simulink model "Quaternions_Method_merge"  (R2021b)
settings: Solver=VariableStepAuto  StartTime=0.0  StopTime=Time  FixedStep=1e-1  RelTol=1e-13  AbsTol=1e-8
values from neighbouring files (symbols this model uses):
  a = 8.6251e+06    (= 8625100)    [Main.m]    (also in main_code.m)
  A_rw = [1 0 0 1/sqrt(3);         0 1 0 1/sqrt(3) ... (first row only)    [Main.m]    (also in main_code.m)
  A_rw_star = [5/6 -1/6 -1/6;              -1/6  5/6 -1/6 ... (first row only)    [Main.m]    (also in main_code.m)
  c = 299792*10^3    (= 299792000)    [Main.m]    (also in main_code.m)
  e = 0.1195    [Main.m]    (also in main_code.m)
  f_mag = 5    [Main.m]
  H_0 = sqrt((g_1_0)^2 + (g_1_1)^2 + (h_1_1)^2)    [Main.m]
  i = 0.3815    [Main.m]    (also in main_code.m)
  MB = [2000; 0.3; 1; 0.12].*1e-2    [Main.m]    (also in main_code.m = [1; 0.3; 0.3; 0.3])
  mr = 1.2*1e-4    (= 0.00012)    [Main.m]    (also in main_code.m)
  muP = G*Mt    (= 398527110340000)    [Main.m]
  omega_0 = [om_x, om_y, om_z]    [Main.m]    (also in main_code.m = [w_0x; w_0y; w_0z])
  p_acc = deg2rad(5)    [Main.m]
  RD = 0.1*ones(1,10)    [Main.m]
  RS_MB = 0.5    [Main.m]
  RS_SP = 0.1    [Main.m]
  sig_b = sig_b^2    [Main.m]    (also in main_code.m)
  sig_n = 0.15*pi/180/3600/sqrt(t_sample)    [Main.m]    (also in main_code.m)
  SP = [2000; 0.3; 1; 0.12].*1e-2    [Main.m]    (also in main_code.m = [3; 0.3; 1; 0.1])
  T = 2*pi/n    [Main.m]    (also in main_code.m = 2*pi / n)
  t_sample = 1/5    (= 0.2)    [Main.m]    (also in main_code.m = 0.1)
  theta0 = 0    [Main.m]
  w_E = (2*pi)/(24*3600)    (= 7.27220521664e-05)    [Main.m]
undefined symbols (not defined in the file or in its folder): magnitude
libraries: matrix_library x14, vrlib x8, simulink x2, simulink_extras x1
(part 2 of 4)

== system Quaternions_Method_merge/Kinematics/Relative_Attitude ==
  A_BN : Inport
  theta : Inport  Port=2
  A_LN : Subsystem
  MatrixMultiply : Product  Multiplication=Matrix(*)
  Transpose : Math  Operator=transpose  SaturateOnIntegerOverflow=on
  A_BL : Outport
  A_L/N : Outport  Port=2
  wires:
  Transpose/1 -> MatrixMultiply/2
  MatrixMultiply/1 -> A_BL/1  "A_BL"
  A_LN/1(A_LN) -> Transpose/1, A_L/N/1
  A_BN/1 -> MatrixMultiply/1
  theta/1 -> A_LN/1(theta)

== system Quaternions_Method_merge/Sensors/Gyroscopes ==
  note: gyro model: STIM300
  omega : Inport
  Integrator : Integrator
  Mux1 : Mux  Inputs=3
  Mux2 : Mux  Inputs=3
  Reshape : Reshape  OutputDimensionality=Column vector (2-D)
  Reshape1 : Reshape  OutputDimensionality=Column vector (2-D)
  Sum : Sum  Inputs=+++
  "b1 " : RandomNumber  Variance=sig_b  Seed=1  SampleTime=t_sample
  b2 : RandomNumber  Variance=sig_b  Seed=2  SampleTime=t_sample
  b3 : RandomNumber  Variance=sig_b  Seed=3  SampleTime=t_sample
  n1 : RandomNumber  Variance=sig_n  Seed=4  SampleTime=t_sample
  n2 : RandomNumber  Variance=sig_n  Seed=5  SampleTime=t_sample
  n3 : RandomNumber  Variance=sig_n  Seed=6  SampleTime=t_sample
  omega_m : Outport
  wires:
  Integrator/1 -> Sum/1
  "b1 "/1 -> Mux1/1
  b2/1 -> Mux1/2
  b3/1 -> Mux1/3
  n3/1 -> Mux2/3
  n2/1 -> Mux2/2
  n1/1 -> Mux2/1
  Mux1/1 -> Reshape/1
  Mux2/1 -> Reshape1/1
  Sum/1 -> omega_m/1
  omega/1 -> Sum/2
  Reshape/1 -> Integrator/1
  Reshape1/1 -> Sum/3

== system Quaternions_Method_merge/Sensors/Magnetometer1 ==
  A_BN : Inport
  b_N : Inport  Port=2
  "Magnetometer " : Subsystem
  b_B computation : Subsystem
  model to reality difference : Subsystem
  b_B : Outport
  wires:
  "Magnetometer "/1(A_BN*_filtered) -> b_B computation/1(A_BN*), model to reality difference/2(A_BN*)
  A_BN/1 -> model to reality difference/1(A_BN), "Magnetometer "/1(A_BN)
  b_N/1 -> b_B computation/2(b_N), model to reality difference/3(b_N)
  b_B computation/1(b_B) -> b_B/1
  "Magnetometer "/2(A_BN*_not_filtered) -> model to reality difference/4(A_BN*1)

== system Quaternions_Method_merge/Sensors/Sun sensor ==
  note: redwire space, digital sun sensor +/- 64°
  S_N : Inport
  A_BN : Inport  Port=2
  Add : Sum  Inputs=+-
  Add1 : Sum  Inputs=+-
  Constant : Constant  Value=0.25*pi/180
  Constant1 : Constant
  Constant2 : Constant  Value=0.25*pi/180
  Constant3 : Constant  Value=0.25*pi/180
  Delay1 : Delay  DelayLength=1
  Discrete Derivative : simulink/Discrete/Discrete Derivative  gainval=T^-1  ICPrevScaledInput=0.0  OutMin=[]  OutMax=[]  OutDataType=fixdt(1, 16)  OutScaling=2^-10  DoSatur=off
  Gain : Gain  Gain=-1
  Gain1 : Gain  Gain=-1
  Gain2 : Gain  Gain=-1
  Matrix Multiply : Product  Multiplication=Matrix(*)
  Matrix Multiply1 : Product  Multiplication=Matrix(*)
  Product : Product
  Product1 : Product
  Product2 : Product
  Random Number : RandomNumber  Variance=0.6*pi/180  SampleTime=1/1000
  Random Number1 : RandomNumber  Variance=0.6*pi/180  SampleTime=1/1000
  Random Number2 : RandomNumber  Variance=0.6*pi/180  SampleTime=1/1000
  Reshape : Reshape  OutputDimensionality=Customize  OutputDimensions=[3,3]
  Scope : Scope
  Vector Concatenate : Concatenate  NumInputs=9
  S_B : Outport
  wires:
  S_N/1 -> Matrix Multiply1/2
  Random Number/1 -> Product/2
  Constant/1 -> Product/1
  Matrix Multiply/1 -> Add1/1
  Discrete Derivative/1 -> Delay1/1
  Add1/1 -> Add/1, Discrete Derivative/1, S_B/1
  Constant1/1 -> Vector Concatenate/8, Vector Concatenate/5, Vector Concatenate/1
  Constant2/1 -> Product1/1
  Random Number1/1 -> Product1/2
  Random Number2/1 -> Product2/2
  Constant3/1 -> Product2/1
  Product2/1 -> Vector Concatenate/4, Gain/1
  Gain/1 -> Vector Concatenate/2
  Product1/1 -> Vector Concatenate/3, Gain2/1
  Gain1/1 -> Vector Concatenate/6
  Product/1 -> Gain1/1, Vector Concatenate/9
  Gain2/1 -> Vector Concatenate/7
  Delay1/1 -> Add1/2
  Reshape/1 -> Matrix Multiply/1
  Vector Concatenate/1 -> Reshape/1
  A_BN/1 -> Matrix Multiply1/1
  Matrix Multiply1/1 -> Add/2, Matrix Multiply/2
  Add/1 -> Scope/1

== system Quaternions_Method_merge/Sun Pointing /Pointing error with DCM ==
  A_B_N from attitude determination : Inport
  S_N : Inport  Port=2
  A_B_N from Euler : Inport  Port=3
  Add : Sum  Inputs=+|-
  Desired attitude : Subsystem
  Detected pointing error : Subsystem
  Real pointing error : Subsystem
  Difference between real and detected pointing error : Outport
  wires:
  A_B_N from attitude determination/1 -> Detected pointing error/2(A_B_N from attitude determination)
  Add/1 -> Difference between real and detected pointing error/1
  A_B_N from Euler/1 -> Real pointing error/1(" A_B_N from Euler")
  Desired attitude/1(Desired A_B_N) -> Real pointing error/2(Desired A_B_N), Detected pointing error/1(Desired A_B_N)
  Detected pointing error/1(detected pointing error) -> Add/2
  Real pointing error/1(real pointing error) -> Add/1
  S_N/1 -> Desired attitude/1(S_N)

== system Quaternions_Method_merge/Sun Pointing /Pointing error with quaternions ==
  A_B_N from attitude determination : Inport
  S_N : Inport  Port=2
  A_B_N from Euler : Inport  Port=3
  Add : Sum  Inputs=+|-
  Add1 : Sum  Inputs=+|-
  Creation of quaternion : Subsystem
  Creation of the quaternion : Subsystem
  Creation quaternion : Subsystem
  Desired attitude : Subsystem
  real pointing error : Outport
  detected pointing error : Outport  Port=2
  wires:
  S_N/1 -> Desired attitude/1(S_N)
  A_B_N from attitude determination/1 -> Creation of the quaternion/1(A_B_N from attitude determination)
  A_B_N from Euler/1 -> Creation of quaternion/1(A_B_N from Euler)
  Desired attitude/1(Desired A_B_N) -> Creation quaternion/1(Desired A_B_N)
  Creation of quaternion/1(q_Att_det) -> Add/1
  Creation quaternion/1(q_des) -> Add1/1, Add/2
  Creation of the quaternion/1(q_Att_det) -> Add1/2
  Add/1 -> real pointing error/1
  Add1/1 -> detected pointing error/1

== system Quaternions_Method_merge/Attitude determination/q to DCM/q_cross ==
  q_vect : Inport
  Demux : Demux  Outputs=3
  Gain : Gain  Gain=-1
  Gain1 : Gain  Gain=-1
  Gain2 : Gain  Gain=-1
  Ground : Ground
  Reshape : Reshape  OutputDimensionality=Customize  OutputDimensions=[3,3]
  Vector Concatenate : Concatenate  NumInputs=9
  q_cross : Outport
  wires:
  q_vect/1 -> Demux/1
  Reshape/1 -> q_cross/1
  Vector Concatenate/1 -> Reshape/1
  Ground/1 -> Vector Concatenate/1, Vector Concatenate/5, Vector Concatenate/9
  Gain/1 -> Vector Concatenate/3
  Gain1/1 -> Vector Concatenate/4
  Gain2/1 -> Vector Concatenate/8
  Demux/1 -> [q1]
  Demux/2 -> [q2]
  Demux/3 -> [q3]
  [q3] -> Vector Concatenate/2
  [q2] -> Gain/1
  [q3] -> Gain1/1
  [q1] -> Vector Concatenate/6
  [q2] -> Vector Concatenate/7
  [q1] -> Gain2/1

== system Quaternions_Method_merge/Enviroment/Magnetic torque /Creation of parasitic torque ==
  Constant : Constant  Value=0.01
  Constant1 : Constant  Value=0.05
  Constant2 : Constant  Value=0.01
  Mux : Mux  Inputs=3
  Reshape : Reshape  OutputDimensionality=Column vector (2-D)
  m : Outport
  wires:
  Constant/1 -> Mux/1
  Constant1/1 -> Mux/2
  Constant2/1 -> Mux/3
  Mux/1 -> Reshape/1
  Reshape/1 -> m/1

== system Quaternions_Method_merge/Enviroment/Magnetic torque /Magnetic torque in body frame ==
  A_B_N : Inport
  r_N : Inport  Port=2
  R : Inport  Port=3
  Add : Sum  Inputs=+++
  Add1 : Sum  Inputs=+|-
  Constant : Constant  Value=3
  Constant1 : Constant  Value=H_0
  Constant2 : Constant  Value=3
  Demux : Demux  Outputs=3
  Direction of M field : Subsystem
  Divide : Product  Inputs=*/
  Dot Product : DotProduct  InputSameDT=on  OutDataTypeStr=Inherit: Inherit via internal rule
  Gain : Gain  Gain=3
  Math Function : Math  Operator=pow  SaturateOnIntegerOverflow=on
  Math Function1 : Math  Operator=magnitude^2  SaturateOnIntegerOverflow=on
  Math Function2 : Math  Operator=magnitude^2  SaturateOnIntegerOverflow=on
  Math Function3 : Math  Operator=magnitude^2  SaturateOnIntegerOverflow=on
  Math Function4 : Math  Operator=pow  SaturateOnIntegerOverflow=on
  MatrixMultiply : Product  Multiplication=Matrix(*)
  Normalize Vector : vrlib/Utilities/Normalize Vector  maxzero=0
  Product : Product
  Product1 : Product
  Product2 : Product
  Reshape : Reshape  OutputDimensionality=Column vector (2-D)
  Sqrt : Sqrt  SaturateOnIntegerOverflow=on
  b_B : Outport
  b_N : Outport  Port=2
  wires:
  Normalize Vector/1 -> Product1/1, Dot Product/1
  Demux/2 -> Math Function2/1
  Constant1/1 -> Product/2
  Constant/1 -> Math Function4/2
  Demux/1 -> Math Function1/1
  MatrixMultiply/1 -> b_B/1
  Math Function1/1 -> Add/1
  Demux/3 -> Math Function3/1
  Divide/1 -> Product2/1
  Add/1 -> Sqrt/1
  Math Function/1 -> Divide/2
  Product1/1 -> Gain/1
  Math Function3/1 -> Add/3
  Product/1 -> Divide/1
  Direction of M field/1(m_vect) -> Add1/2, Dot Product/2
  Math Function4/1 -> Product/1
  Add1/1 -> Product2/2
  Math Function2/1 -> Add/2
  Gain/1 -> Add1/1
  Dot Product/1 -> Product1/2
  Product2/1 -> b_N/1, MatrixMultiply/2  "b_N"
  Sqrt/1 -> Math Function/1
  R/1 -> Math Function4/1
  Reshape/1 -> Demux/1
  r_N/1 -> Reshape/1, Normalize Vector/1
  Constant2/1 -> Math Function/2
  A_B_N/1 -> [A_BN]
  [A_BN] -> MatrixMultiply/1

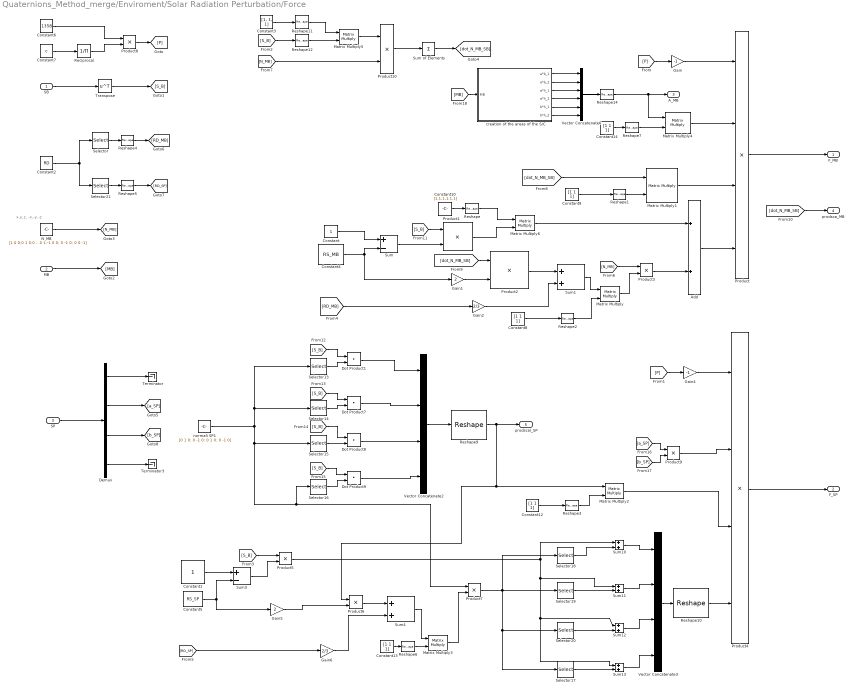
== system Quaternions_Method_merge/Enviroment/Solar Radiation Perturbation/Force ==
  note: x,y,z, -x,-y.-z
  SB : Inport
  MB : Inport  Port=2
  SP : Inport  Port=3
  Add : Sum
  Constant : Constant
  Constant1 : Constant
  Constant10 : Constant  Value=[1,1,1,1,1,1]
  Constant{8..9,12..14} (5 alike) : Constant  Value=[1 1 1]
  Constant2 : Constant  Value=RD
  Constant3 : Constant  Value=[1, 1, 1]
  Constant4 : Constant  Value=RS_MB
  Constant5 : Constant  Value=RS_SP
  Constant6 : Constant  Value=1358
  Constant7 : Constant  Value=c
  Demux : Demux
  Dot Product{1,7..9} (4 alike) : DotProduct  InputSameDT=on  OutDataTypeStr=Inherit: Inherit via internal rule
  Gain : Gain  Gain=-1
  Gain1 : Gain  Gain=2
  Gain2 : Gain  Gain=2/3
  Gain4 : Gain  Gain=-1
  Gain5 : Gain  Gain=2
  Gain6 : Gain  Gain=2/3
  Matrix Multiply{,1..6} (7 alike) : Product  Multiplication=Matrix(*)
  N_MB : Constant  Value=[1 0 0;0 1 0;0 0 1;-1 0 0; 0 -1 0; 0 0 -1]
  Product : Product  Inputs=4
  Product{1..3,5..10} (9 alike) : Product
  Product4 : Product  Inputs=4
  Reciprocal : Product  Inputs=/
  Reshape{,4..5,12,14} (5 alike) : Reshape  OutputDimensionality=Column vector (2-D)
  Reshape{1..3,6..7,11} (6 alike) : Reshape  OutputDimensionality=Row vector (2-D)
  Reshape10 : Reshape  OutputDimensionality=Customize  OutputDimensions=[4,3]
  Reshape9 : Reshape  OutputDimensionality=Customize  OutputDimensions=[4,1]
  Selector : Selector  InputPortWidth=10  IndexOptions=Index vector (dialog)  Indices=[1 2 3 4 5 6]  OutputSizes=1
  Selector13 : Selector  NumberOfDimensions=2  InputPortWidth=3  IndexOptions=Index vector (dialog),Index vector (dialog)  Indices=1,[1 2 3]  OutputSizes=1,1
  Selector14 : Selector  NumberOfDimensions=2  InputPortWidth=3  IndexOptions=Index vector (dialog),Index vector (dialog)  Indices=2,[1 2 3]  OutputSizes=1,1
  Selector15 : Selector  NumberOfDimensions=2  InputPortWidth=3  IndexOptions=Index vector (dialog),Index vector (dialog)  Indices=3,[1 2 3]  OutputSizes=1,1
  Selector16 : Selector  NumberOfDimensions=2  InputPortWidth=3  IndexOptions=Index vector (dialog),Index vector (dialog)  Indices=4,[1 2 3]  OutputSizes=1,1
  Selector17 : Selector  NumberOfDimensions=2  InputPortWidth=3  IndexOptions=Index vector (dialog),Index vector (dialog)  Indices=4,[1 2 3]  OutputSizes=1,1
  Selector18 : Selector  NumberOfDimensions=2  InputPortWidth=3  IndexOptions=Index vector (dialog),Index vector (dialog)  Indices=1,[1 2 3]  OutputSizes=1,1
  Selector19 : Selector  NumberOfDimensions=2  InputPortWidth=3  IndexOptions=Index vector (dialog),Index vector (dialog)  Indices=2,[1 2 3]  OutputSizes=1,1
  Selector20 : Selector  NumberOfDimensions=2  InputPortWidth=3  IndexOptions=Index vector (dialog),Index vector (dialog)  Indices=3,[1 2 3]  OutputSizes=1,1
  Selector21 : Selector  InputPortWidth=10  IndexOptions=Index vector (dialog)  Indices=[7 8 9 10]  OutputSizes=1
  Sum : Sum  Inputs=+-
  Sum of Elements : Sum  Inputs=+  CollapseMode=Specified dimension  CollapseDim=2
  Sum1 : Sum
  Sum{10..13} (4 alike) : Sum  Inputs=|+|+|
  Sum3 : Sum  Inputs=+-
  Sum4 : Sum
  Terminator : Terminator
  Terminator3 : Terminator
  Transpose : Math  Operator=transpose  SaturateOnIntegerOverflow=on
  Vector Concatenate2 : Concatenate  NumInputs=4
  Vector Concatenate3 : Concatenate  NumInputs=4
  Vector Concatenate6 : Concatenate  NumInputs=6
  creation of the areas of the S/C : Subsystem
  normali SP1 : Constant  Value=[0 1 0; 0 -1 0; 0 1 0; 0 -1 0]
  F_MB : Outport
  F_SP : Outport  Port=2
  A_MB : Outport  Port=3
  prodsca_MB : Outport  Port=4
  prodscal_SP : Outport  Port=5
  wires:
  Gain/1 -> Product/1
  Reshape9/1 -> prodscal_SP/1, Product6/1, Matrix Multiply2/1
  Gain5/1 -> Product6/2
  Constant1/1 -> Sum3/1
  Gain1/1 -> Product2/2
  Reshape5/1 -> [RD_SP]
  SB/1 -> Transpose/1
  Add/1 -> Product/4
  Gain6/1 -> Sum4/2
  Gain4/1 -> Product4/1
  [P] -> Gain/1
  Reshape4/1 -> [RD_MB]
  Sum3/1 -> Product5/2
  Product6/1 -> Sum4/1
  Constant5/1 -> Sum3/2, Gain5/1
  Product2/1 -> Sum1/1
  [RD_MB] -> Gain2/1
  Gain2/1 -> Sum1/2
  Constant/1 -> Sum/1
  Constant4/1 -> Sum/2, Gain1/1
  Sum/1 -> Product1/2
  Product/1 -> F_MB/1
  [P] -> Gain4/1
  [RD_SP] -> Gain6/1
  Constant6/1 -> Product8/1
  Product8/1 -> [P]
  [S_B] -> Product1/1
  Constant8/1 -> Reshape2/1
  Reshape2/1 -> Matrix Multiply/2
  Sum1/1 -> Matrix Multiply/1
  Matrix Multiply/1 -> Product3/2
  Constant9/1 -> Reshape1/1
  Reshape1/1 -> Matrix Multiply1/2
  Matrix Multiply1/1 -> Product/3
  Transpose/1 -> [S_B]
  Selector14/1 -> Dot Product7/2
  [S_B] -> Dot Product8/1
  Selector15/1 -> Dot Product8/2
  Selector16/1 -> Dot Product9/2
  [S_B] -> Dot Product7/1
  [S_B] -> Dot Product1/1
  Dot Product8/1 -> Vector Concatenate2/3
  Dot Product7/1 -> Vector Concatenate2/2
  Dot Product1/1 -> Vector Concatenate2/1
  Dot Product9/1 -> Vector Concatenate2/4
  Selector13/1 -> Dot Product1/2
  normali SP1/1 -> Product7/1, Selector16/1, Selector15/1, Selector13/1, Selector14/1
  [S_B] -> Dot Product9/1
  Reshape3/1 -> Matrix Multiply2/2
  Constant12/1 -> Reshape3/1
  Matrix Multiply2/1 -> Product4/3
  [S_B] -> Product5/1
  Constant13/1 -> Reshape6/1
  Reshape6/1 -> Matrix Multiply3/2
  Sum4/1 -> Matrix Multiply3/1
  Matrix Multiply3/1 -> Product7/2
  Selector20/1 -> Sum12/2
  Sum13/1 -> Vector Concatenate3/4
  Selector19/1 -> Sum11/2
  Selector18/1 -> Sum10/2
  Sum10/1 -> Vector Concatenate3/1
  Sum12/1 -> Vector Concatenate3/3
  Sum11/1 -> Vector Concatenate3/2
  Product7/1 -> Selector17/1, Selector20/1, Selector18/1, Selector19/1
  Selector17/1 -> Sum13/2
  Product5/1 -> Sum10/1, Sum11/1, Sum13/1, Sum12/1
  Reshape10/1 -> Product4/4
  Reshape7/1 -> Matrix Multiply4/2
  Constant14/1 -> Reshape7/1
  Matrix Multiply4/1 -> Product/2
  Reciprocal/1 -> Product8/2
  Constant7/1 -> Reciprocal/1
  Vector Concatenate2/1 -> Reshape9/1
  Vector Concatenate3/1 -> Reshape10/1
  Product4/1 -> F_SP/1
  Vector Concatenate6/1 -> Reshape14/1
  creation of the areas of the S/C/1(a*b_1) -> Vector Concatenate6/1
  creation of the areas of the S/C/2(a*b_2) -> Vector Concatenate6/2
  creation of the areas of the S/C/3(a*h_1) -> Vector Concatenate6/3
  creation of the areas of the S/C/4(a*h_2) -> Vector Concatenate6/4
  creation of the areas of the S/C/5(b*h_1) -> Vector Concatenate6/5
  creation of the areas of the S/C/6(b*h_2) -> Vector Concatenate6/6
  Reshape14/1 -> A_MB/1, Matrix Multiply4/1
  MB/1 -> [MB]
  SP/1 -> Demux/1
  Demux/2 -> [a_SP]
  Demux/4 -> Terminator3/1
  Demux/3 -> [b_SP]
  Demux/1 -> Terminator/1
  [a_SP] -> Product9/1
  [b_SP] -> Product9/2
  Product9/1 -> Product4/2
  Selector/1 -> Reshape4/1
  Selector21/1 -> Reshape5/1
  Constant2/1 -> Selector21/1, Selector/1
  [MB] -> creation of the areas of the S/C/1(MB)
  Constant3/1 -> Reshape11/1
  Reshape11/1 -> Matrix Multiply5/1
  Matrix Multiply5/1 -> Product10/1
  Product10/1 -> Sum of Elements/1
  [S_B] -> Reshape12/1
  Reshape12/1 -> Matrix Multiply5/2
  N_MB/1 -> [N_MB]
  [N_MB] -> Product3/1
  [N_MB] -> Product10/2
  Sum of Elements/1 -> [dot_N_MB_SB]
  [dot_N_MB_SB] -> Matrix Multiply1/1
  [dot_N_MB_SB] -> Product2/1
  Constant10/1 -> Reshape/1
  Reshape/1 -> Matrix Multiply6/1
  Product1/1 -> Matrix Multiply6/2
  Matrix Multiply6/1 -> Add/1
  Product3/1 -> Add/2
  [dot_N_MB_SB] -> prodsca_MB/1

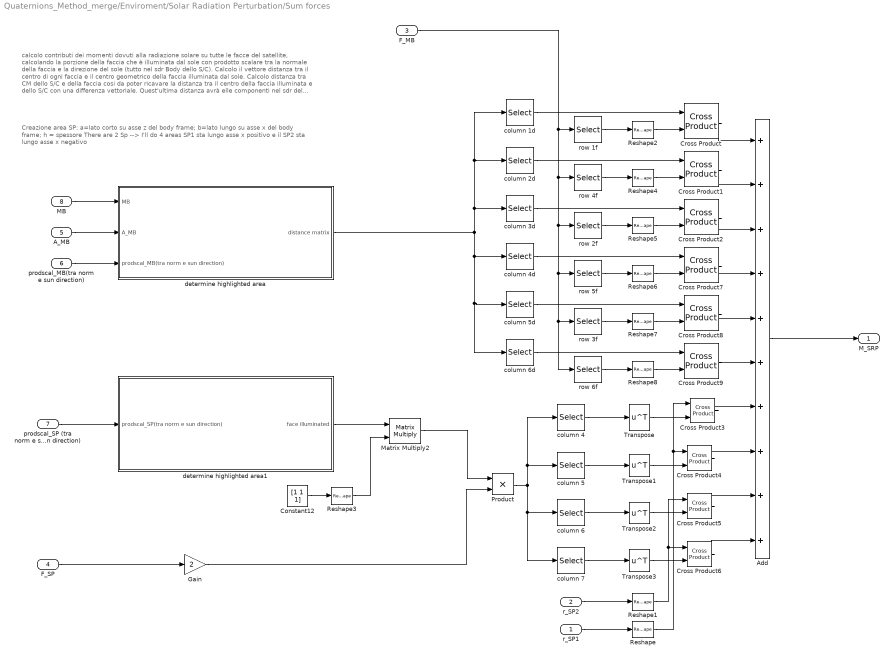
== system Quaternions_Method_merge/Enviroment/Solar Radiation Perturbation/Sum forces ==
  note: Creazione area SP: a=lato corto su asse z del body frame; b=lato lungo su asse x del body frame; h = spessore
      | There are 2 Sp --> I'll do 4 areas
      | SP1 sta lungo asse x positivo e il SP2 sta lungo asse x negativo
  note: calcolo contributi dei momenti dovuti alla radiazione solare su tutte le facce del satellite, calcolando la porzione della faccia che è illuminata dal sole con prodotto scalare tra la normale della faccia e la direzione del sole (tutto nel sdr Body dello S/C). Calcolo il vettore distanza tra il centro di ogni faccia e il centro geometrico della faccia illuminata dal sole. Calcolo distanza tra CM dello S/C e della faccia cosi da poter ricavare la distanza tra il centro della faccia illuminata e dello S/C con una differenza vettoriale. Quest'ultima distanza avrà elle componenti nel sdr del S/C (body)
  r_SP1 : Inport
  r_SP2 : Inport  Port=2
  F_MB : Inport  Port=3
  F_SP : Inport  Port=4
  A_MB : Inport  Port=5
  prodscal_MB(tra norm e sun direction) : Inport  Port=6
  prodscal_SP (tra norm e sun direction) : Inport  Port=7
  MB : Inport  Port=8
  Add : Sum  Inputs=+|+|+|+|+|+|+|+|+|+
  Constant12 : Constant  Value=[1 1 1]
  Cross Product{,1..9} (10 alike) : matrix_library/Cross Product
      settings: SourceProductBaseCode=SL
  Gain : Gain  Gain=2
  Matrix Multiply2 : Product  Multiplication=Matrix(*)
  Product : Product
  Reshape{,1..2,4..8} (8 alike) : Reshape  OutputDimensionality=Column vector (2-D)
  Reshape3 : Reshape  OutputDimensionality=Row vector (2-D)
  Transpose{,1..3} (4 alike) : Math  Operator=transpose  SaturateOnIntegerOverflow=on
  column 1d : Selector  NumberOfDimensions=2  InputPortWidth=3  IndexOptions=Index vector (dialog),Index vector (dialog)  Indices=[1 2 3],1  OutputSizes=1,1
  column 2d : Selector  NumberOfDimensions=2  InputPortWidth=3  IndexOptions=Index vector (dialog),Index vector (dialog)  Indices=[1 2 3],2  OutputSizes=1,1
  column 3d : Selector  NumberOfDimensions=2  InputPortWidth=3  IndexOptions=Index vector (dialog),Index vector (dialog)  Indices=[1 2 3],3  OutputSizes=1,1
  column 4 : Selector  NumberOfDimensions=2  InputPortWidth=3  IndexOptions=Index vector (dialog),Index vector (dialog)  Indices=1,[1 2 3]  OutputSizes=1,1
  column 4d : Selector  NumberOfDimensions=2  InputPortWidth=3  IndexOptions=Index vector (dialog),Index vector (dialog)  Indices=[1 2 3],1  OutputSizes=1,1
  column 5 : Selector  NumberOfDimensions=2  InputPortWidth=3  IndexOptions=Index vector (dialog),Index vector (dialog)  Indices=2,[1 2 3]  OutputSizes=1,1
  column 5d : Selector  NumberOfDimensions=2  InputPortWidth=3  IndexOptions=Index vector (dialog),Index vector (dialog)  Indices=[1 2 3],2  OutputSizes=1,1
  column 6 : Selector  NumberOfDimensions=2  InputPortWidth=3  IndexOptions=Index vector (dialog),Index vector (dialog)  Indices=3,[1 2 3]  OutputSizes=1,1
  column 6d : Selector  NumberOfDimensions=2  InputPortWidth=3  IndexOptions=Index vector (dialog),Index vector (dialog)  Indices=[1 2 3],3  OutputSizes=1,1
  column 7 : Selector  NumberOfDimensions=2  InputPortWidth=3  IndexOptions=Index vector (dialog),Index vector (dialog)  Indices=4,[1 2 3]  OutputSizes=1,1
  determine highlighted area : Subsystem
  determine highlighted area1 : Subsystem
  row 1f : Selector  NumberOfDimensions=2  InputPortWidth=3  IndexOptions=Index vector (dialog),Index vector (dialog)  Indices=1,[1 2 3]  OutputSizes=1,1
  row 2f : Selector  NumberOfDimensions=2  InputPortWidth=3  IndexOptions=Index vector (dialog),Index vector (dialog)  Indices=2,[1 2 3]  OutputSizes=1,1
  row 3f : Selector  NumberOfDimensions=2  InputPortWidth=3  IndexOptions=Index vector (dialog),Index vector (dialog)  Indices=3,[1 2 3]  OutputSizes=1,1
  row 4f : Selector  NumberOfDimensions=2  InputPortWidth=3  IndexOptions=Index vector (dialog),Index vector (dialog)  Indices=4,[1 2 3]  OutputSizes=1,1
  row 5f : Selector  NumberOfDimensions=2  InputPortWidth=3  IndexOptions=Index vector (dialog),Index vector (dialog)  Indices=5,[1 2 3]  OutputSizes=1,1
  row 6f : Selector  NumberOfDimensions=2  InputPortWidth=3  IndexOptions=Index vector (dialog),Index vector (dialog)  Indices=6,[1 2 3]  OutputSizes=1,1
  M_SRP : Outport
  wires:
  prodscal_MB(tra norm e sun direction)/1 -> determine highlighted area/3(prodscal_MB(tra norm e sun direction))
  Add/1 -> M_SRP/1
  A_MB/1 -> determine highlighted area/2(A_MB)
  column 2d/1 -> Cross Product1/1
  column 1d/1 -> Cross Product/1
  column 3d/1 -> Cross Product2/1
  Cross Product1/1 -> Add/2
  Cross Product/1 -> Add/1
  Cross Product2/1 -> Add/3
  prodscal_SP (tra norm e sun direction)/1 -> determine highlighted area1/1(prodscal_SP(tra norm e sun direction))
  F_SP/1 -> Gain/1
  Gain/1 -> Product/2
  Reshape3/1 -> Matrix Multiply2/2
  Constant12/1 -> Reshape3/1
  determine highlighted area1/1(face illuminated) -> Matrix Multiply2/1
  Matrix Multiply2/1 -> Product/1
  r_SP1/1 -> Reshape/1
  r_SP2/1 -> Reshape1/1
  Product/1 -> column 7/1, column 6/1, column 4/1, column 5/1
  Cross Product3/1 -> Add/7
  Cross Product4/1 -> Add/8
  Cross Product5/1 -> Add/9
  Cross Product6/1 -> Add/10
  column 4/1 -> Transpose/1
  column 5/1 -> Transpose1/1
  column 6/1 -> Transpose2/1
  column 7/1 -> Transpose3/1
  Reshape/1 -> Cross Product3/1, Cross Product4/1
  Reshape1/1 -> Cross Product5/1, Cross Product6/1
  Transpose/1 -> Cross Product3/2
  Transpose1/1 -> Cross Product4/2
  Transpose2/1 -> Cross Product5/2
  Transpose3/1 -> Cross Product6/2
  Cross Product9/1 -> Add/6
  Cross Product7/1 -> Add/4
  Cross Product8/1 -> Add/5
  column 6d/1 -> Cross Product9/1
  column 4d/1 -> Cross Product7/1
  column 5d/1 -> Cross Product8/1
  determine highlighted area/1(distance matrix) -> column 2d/1, column 1d/1, column 3d/1, column 6d/1, column 5d/1, column 4d/1
  row 1f/1 -> Reshape2/1
  row 4f/1 -> Reshape4/1
  row 2f/1 -> Reshape5/1
  row 5f/1 -> Reshape6/1
  row 3f/1 -> Reshape7/1
  row 6f/1 -> Reshape8/1
  F_MB/1 -> row 6f/1, row 3f/1, row 5f/1, row 2f/1, row 4f/1, row 1f/1
  Reshape2/1 -> Cross Product/2
  Reshape4/1 -> Cross Product1/2
  Reshape5/1 -> Cross Product2/2
  Reshape6/1 -> Cross Product7/2
  Reshape7/1 -> Cross Product8/2
  Reshape8/1 -> Cross Product9/2
  MB/1 -> determine highlighted area/1(MB)

== system Quaternions_Method_merge/Enviroment/Solar Radiation Perturbation/Sun position body ==
  A_B_N : Inport
  Clock : Clock
  Constant : Constant  Value=2*pi
  Constant1 : Constant  Value=365*24*60*60
  Constant2 : Constant  Value=23.45
  Degrees to Radians : simulink_extras/Transformations/Degrees to Radians
  MatrixMultiply : Product  Multiplication=Matrix(*)
  Mux : Mux  Inputs=3
  Product{,1..3} (4 alike) : Product
  Reciprocal : Product  Inputs=1
  Reshape : Reshape  OutputDimensionality=Column vector (2-D)
  Sin : Trigonometry  Operator=cos
  Sin1 : Trigonometry
  Sin2 : Trigonometry  Operator=cos
  Sin3 : Trigonometry
  S_B : Outport
  S_N : Outport  Port=2
  wires:
  Product3/1 -> Mux/3
  Degrees to Radians/1 -> Sin3/1, Sin2/1
  Constant1/1 -> Reciprocal/1
  Sin2/1 -> Product2/2
  Product/1 -> Product1/1  "n"
  Constant2/1 -> Degrees to Radians/1
  Product1/1 -> Sin/1, Sin1/1  "n*t"
  Product2/1 -> Mux/2
  Sin3/1 -> Product3/2
  Clock/1 -> Product1/2
  Sin1/1 -> Product3/1, Product2/1
  Constant/1 -> Product/1
  Sin/1 -> Mux/1
  Reciprocal/1 -> Product/2
  Mux/1 -> Reshape/1
  A_B_N/1 -> MatrixMultiply/1
  MatrixMultiply/1 -> S_B/1
  Reshape/1 -> S_N/1, MatrixMultiply/2

== system Quaternions_Method_merge/Kinematics/Creazione Matrice A_BN/column 1 ==
  q_normalizzato : Inport
  Demux : Demux
  Gain : Gain  Gain=2
  Gain1 : Gain  Gain=2
  Mux : Mux  Inputs=3
  Product{,1..3} (4 alike) : Product
  Square{,1..3} (4 alike) : Math  Operator=square  SaturateOnIntegerOverflow=on
  Sum : Sum  Inputs=|+|-|-|+|
  Sum1 : Sum  Inputs=|+|-|
  Sum2 : Sum  Inputs=|+|+|
  Column 1 : Outport
  wires:
  Demux/4 -> [q4]
  Demux/1 -> [q1]
  q_normalizzato/1 -> Demux/1
  Demux/3 -> [q3]
  Demux/2 -> [q2]
  [q1] -> Square/1
  [q2] -> Square3/1
  [q3] -> Square2/1
  [q4] -> Square1/1
  Square3/1 -> Sum/2
  Square/1 -> Sum/1
  Square1/1 -> Sum/4
  Square2/1 -> Sum/3
  [q4] -> Product1/2
  [q1] -> Product/1
  [q2] -> Product/2
  [q3] -> Product1/1
  Product/1 -> Sum1/1
  Product1/1 -> Sum1/2
  Sum1/1 -> Gain/1
  [q4] -> Product3/2
  [q1] -> Product2/1
  Product3/1 -> Sum2/2
  Product2/1 -> Sum2/1
  Sum2/1 -> Gain1/1
  [q3] -> Product2/2
  [q2] -> Product3/1
  Sum/1 -> Mux/1
  Gain/1 -> Mux/2
  Gain1/1 -> Mux/3
  Mux/1 -> Column 1/1

== system Quaternions_Method_merge/Kinematics/Creazione Matrice A_BN/column 2 ==
  q_normalizzato : Inport
  Demux : Demux
  Gain : Gain  Gain=2
  Gain1 : Gain  Gain=2
  Mux : Mux  Inputs=3
  Product{,1..3} (4 alike) : Product
  Square{,1..3} (4 alike) : Math  Operator=square  SaturateOnIntegerOverflow=on
  Sum : Sum  Inputs=|-|+|-|+|
  Sum1 : Sum  Inputs=|+|+|
  Sum2 : Sum  Inputs=|+|-|
  Column 2 : Outport
  wires:
  Demux/4 -> [q4]
  Demux/1 -> [q1]
  q_normalizzato/1 -> Demux/1
  Demux/3 -> [q3]
  Demux/2 -> [q2]
  Mux/1 -> Column 2/1
  Gain1/1 -> Mux/3
  Product2/1 -> Sum2/1
  Product3/1 -> Sum2/2
  Sum2/1 -> Gain1/1
  Sum1/1 -> Gain/1
  [q2] -> Product/2
  [q3] -> Product1/1
  [q4] -> Product1/2
  Product/1 -> Sum1/1
  Gain/1 -> Mux/1
  [q1] -> Product/1
  Product1/1 -> Sum1/2
  Sum/1 -> Mux/2
  [q1] -> Square/1
  Square1/1 -> Sum/4
  Square3/1 -> Sum/2
  [q4] -> Square1/1
  Square2/1 -> Sum/3
  [q2] -> Square3/1
  [q3] -> Square2/1
  Square/1 -> Sum/1
  [q2] -> Product2/1
  [q3] -> Product2/2
  [q1] -> Product3/1
  [q4] -> Product3/2

== system Quaternions_Method_merge/Kinematics/Creazione Matrice A_BN/column 3 ==
  q_normalizzato : Inport
  Demux : Demux
  Gain : Gain  Gain=2
  Gain1 : Gain  Gain=2
  Mux : Mux  Inputs=3
  Product{,1..3} (4 alike) : Product
  Square{,1..3} (4 alike) : Math  Operator=square  SaturateOnIntegerOverflow=on
  Sum : Sum  Inputs=|-|-|+|+|
  Sum1 : Sum  Inputs=|+|-|
  Sum2 : Sum  Inputs=|+|+|
  Column 3 : Outport
  wires:
  Demux/4 -> [q4]
  Demux/1 -> [q1]
  q_normalizzato/1 -> Demux/1
  Demux/3 -> [q3]
  Demux/2 -> [q2]
  Gain/1 -> Mux/1
  Product1/1 -> Sum1/2
  [q4] -> Product1/2
  Product/1 -> Sum1/1
  Mux/1 -> Column 3/1
  [q1] -> Product/1
  Sum1/1 -> Gain/1
  [q1] -> Square/1
  Square2/1 -> Sum/3
  Square3/1 -> Sum/2
  [q4] -> Square1/1
  Square1/1 -> Sum/4
  Square/1 -> Sum/1
  Sum/1 -> Mux/3
  [q3] -> Square2/1
  [q2] -> Square3/1
  [q2] -> Product2/1
  Product3/1 -> Sum2/2
  Gain1/1 -> Mux/2
  Sum2/1 -> Gain1/1
  Product2/1 -> Sum2/1
  [q3] -> Product2/2
  [q4] -> Product3/2
  [q1] -> Product3/1
  [q3] -> Product/2
  [q2] -> Product1/1

== system Quaternions_Method_merge/Kinematics/Creazione quaternione/Initial condition quaternion ==
  A_LN : Inport
  Constant : Constant
  Demux1 : Demux  Outputs=9
  Divide : Product  Inputs=*/
  Divide1 : Product  Inputs=*/
  Divide2 : Product  Inputs=*/
  Gain : Gain  Gain=0.5
  Gain1 : Gain  Gain=4
  Gain2 : Gain  Gain=4
  Gain3 : Gain  Gain=4
  Mux : Mux
  Reshape : Reshape  OutputDimensionality=Column vector (2-D)
  Reshape1 : Reshape  OutputDimensionality=Column vector (2-D)
  Square Root : Sqrt  SaturateOnIntegerOverflow=on
  Sum : Sum  Inputs=|+|+|+|+|
  Sum1 : Sum  Inputs=|+|-|
  Sum2 : Sum  Inputs=|+|-|
  Sum3 : Sum  Inputs=|+|-|
  Output : Outport
  wires:
  Demux1/3 -> [A31]
  Demux1/9 -> [A33]
  Demux1/1 -> [A11]
  A_LN/1 -> Reshape1/1
  Reshape1/1 -> Demux1/1
  Demux1/5 -> [A22]
  Demux1/2 -> [A21]
  Demux1/4 -> [A12]
  Demux1/6 -> [A32]
  Demux1/7 -> [A13]
  Demux1/8 -> [A23]
  Constant/1 -> Sum/1
  [A11] -> Sum/2
  [A22] -> Sum/3
  [A33] -> Sum/4
  Sum/1 -> Square Root/1
  Square Root/1 -> Gain/1
  Gain/1 -> Mux/4, [q4]
  [A23] -> Sum1/1
  [A32] -> Sum1/2
  Sum1/1 -> Divide/1
  [q4] -> Gain1/1
  Gain1/1 -> Divide/2
  Divide/1 -> Mux/1
  Divide1/1 -> Mux/2
  [A31] -> Sum2/1
  [A13] -> Sum2/2
  Sum2/1 -> Divide1/1
  [q4] -> Gain2/1
  Gain2/1 -> Divide1/2
  Divide2/1 -> Mux/3
  [A12] -> Sum3/1
  [A21] -> Sum3/2
  Sum3/1 -> Divide2/1
  [q4] -> Gain3/1
  Gain3/1 -> Divide2/2
  Mux/1 -> Reshape/1
  Reshape/1 -> Output/1

== system Quaternions_Method_merge/Kinematics/Creazione quaternione/Normalisation ==
  In1 : Inport
  Normalize Vector : vrlib/Utilities/Normalize Vector  maxzero=0
  Reshape : Reshape  OutputDimensionality=Column vector (2-D)
  Out1 : Outport
  wires:
  In1/1 -> Normalize Vector/1
  Normalize Vector/1 -> Reshape/1
  Reshape/1 -> Out1/1

== system Quaternions_Method_merge/Kinematics/Creazione quaternione/Subsystem ==
  om_x : Inport
  om_y : Inport  Port=2
  om_z : Inport  Port=3
  Gain{,1..5} (6 alike) : Gain  Gain=-1
  Ground : Ground
  Reshape : Reshape  OutputDimensionality=Customize  OutputDimensions=[4,4]
  Vector Concatenate : Concatenate  NumInputs=16
  OMEGA1 : Outport
  wires:
  om_y/1 -> Gain3/1, Gain4/1, Vector Concatenate/3, Vector Concatenate/14
  Gain/1 -> Vector Concatenate/2
  om_x/1 -> Gain1/1, Gain2/1, Vector Concatenate/10, Vector Concatenate/13
  Gain1/1 -> Vector Concatenate/4
  om_z/1 -> Gain5/1, Vector Concatenate/15, Gain/1, Vector Concatenate/5
  Reshape/1 -> OMEGA1/1
  Ground/1 -> Vector Concatenate/16, Vector Concatenate/11, Vector Concatenate/6, Vector Concatenate/1
  Gain3/1 -> Vector Concatenate/8
  Gain2/1 -> Vector Concatenate/7
  Gain5/1 -> Vector Concatenate/12
  Vector Concatenate/1 -> Reshape/1
  Gain4/1 -> Vector Concatenate/9

== system Quaternions_Method_merge/Kinematics/Orbit Propagation/vector ==
  theta : Inport
  Constant : Constant  Value=i
  Cos : Trigonometry  Operator=cos
  Cos1 : Trigonometry
  Cos2 : Trigonometry  Operator=cos
  Cos3 : Trigonometry
  Cos4 : Trigonometry
  Mux : Mux  Inputs=3
  Product : Product
  Product1 : Product
  Vector : Outport
  wires:
  Mux/1 -> Vector/1
  Cos/1 -> Mux/1
  Cos1/1 -> Product/1
  Cos2/1 -> Product/2
  Product/1 -> Mux/2
  Cos4/1 -> Product1/2
  Product1/1 -> Mux/3
  Cos3/1 -> Product1/1
  theta/1 -> Cos3/1, Cos1/1, Cos/1
  Constant/1 -> Cos4/1, Cos2/1

== system Quaternions_Method_merge/Kinematics/Relative_Attitude/A_LN ==
  theta : Inport
  Constant : Constant  Value=i
  M1 : Subsystem
  M2 : Subsystem
  MatrixMultiply : Product  Multiplication=Matrix(*)
  A_LN : Outport
  wires:
  theta/1 -> M1/1(Input)
  M1/1(Out1) -> MatrixMultiply/1
  M2/1(Out1) -> MatrixMultiply/2
  MatrixMultiply/1 -> A_LN/1
  Constant/1 -> M2/1(ii)

== system Quaternions_Method_merge/Sensors/Magnetometer1/Magnetometer  ==
  note: Questo blocco serve a verificare ortonrmalizzazione. Per verificare la amtrice in display deve avere daigonale 1
  A_BN : Inport
  Error Matrices : Subsystem
  Matrix Multiply : Product  Inputs=4  Multiplication=Matrix(*)
  RC Low Pass FIlter : Subsystem
  orthonormalization step 1 : Subsystem
  orthonormalization step 2 : Subsystem
  orthonormalization step 3 : Subsystem
  A_BN*_filtered : Outport
  A_BN*_not_filtered : Outport  Port=2
  wires:
  A_BN/1 -> Matrix Multiply/1
  Matrix Multiply/1 -> A_BN*_not_filtered/1, RC Low Pass FIlter/1(A*)
  Error Matrices/1(A_no) -> Matrix Multiply/2
  Error Matrices/2(A_sf) -> Matrix Multiply/3
  Error Matrices/3(A_noise) -> Matrix Multiply/4
  orthonormalization step 1/1(A_BN*_filtered) -> orthonormalization step 2/1(A*(t))
  RC Low Pass FIlter/1(A*_filtered) -> orthonormalization step 1/1(A*(t))
  orthonormalization step 2/1(A_BN*_filtered) -> orthonormalization step 3/1(A*(t))
  orthonormalization step 3/1(A_BN*_filtered) -> A_BN*_filtered/1

== system Quaternions_Method_merge/Sensors/Magnetometer1/b_B computation ==
  A_BN* : Inport
  b_N : Inport  Port=2
  Matrix Multiply : Product  Multiplication=Matrix(*)
  Saturation : Subsystem
  b_B : Outport
  wires:
  A_BN*/1 -> Matrix Multiply/1
  b_N/1 -> Matrix Multiply/2
  Matrix Multiply/1 -> Saturation/1(b_B)
  Saturation/1(b_B saturated) -> b_B/1

== system Quaternions_Method_merge/Sensors/Magnetometer1/model to reality difference ==
  A_BN : Inport
  A_BN* : Inport  Port=2
  b_N : Inport  Port=3
  A_BN*1 : Inport  Port=4
  A_BN1 : InportShadow
  MatrixMultiply{,1..3} (4 alike) : Product  Multiplication=Matrix(*)
  Scope : Scope  NumInputPorts=2
  Sum : Sum  Inputs=|-|+|
  Sum1 : Sum  Inputs=|-|+|
  b_N1 : InportShadow  Port=3
  wires:
  A_BN*/1 -> MatrixMultiply/1
  b_N/1 -> MatrixMultiply1/2, MatrixMultiply/2
  A_BN/1 -> MatrixMultiply1/1
  MatrixMultiply1/1 -> Sum/1
  MatrixMultiply/1 -> Sum/2
  Sum/1 -> Scope/1
  Sum1/1 -> Scope/2
  A_BN1/1 -> MatrixMultiply3/1
  MatrixMultiply3/1 -> Sum1/1
  A_BN*1/1 -> MatrixMultiply2/1
  MatrixMultiply2/1 -> Sum1/2
  b_N1/1 -> MatrixMultiply3/2, MatrixMultiply2/2

== system Quaternions_Method_merge/Sun Pointing /Pointing error with DCM/Desired attitude ==
  S_N : Inport
  Constant : Constant  Value=0
  Constant1 : Constant  Value=0
  Constant2 : Constant
  Cross Product : matrix_library/Cross Product
      settings: SourceProductBaseCode=SL
  Mux : Mux  Inputs=3
  Reshape : Reshape  OutputDimensionality=Column vector (2-D)
  Reshape1 : Reshape  OutputDimensionality=Customize  OutputDimensions=[3,3]
  Transpose : Math  Operator=transpose  SaturateOnIntegerOverflow=on
  Vector Concatenate : Concatenate  NumInputs=3
  Desired A_B_N : Outport
  wires:
  Constant/1 -> Mux/1
  Constant1/1 -> Mux/2
  Constant2/1 -> Mux/3
  Mux/1 -> Reshape/1
  Reshape/1 -> Vector Concatenate/3, Cross Product/1
  S_N/1 -> Cross Product/2, Vector Concatenate/2
  Cross Product/1 -> Vector Concatenate/1
  Vector Concatenate/1 -> Reshape1/1
  Reshape1/1 -> Transpose/1
  Transpose/1 -> Desired A_B_N/1

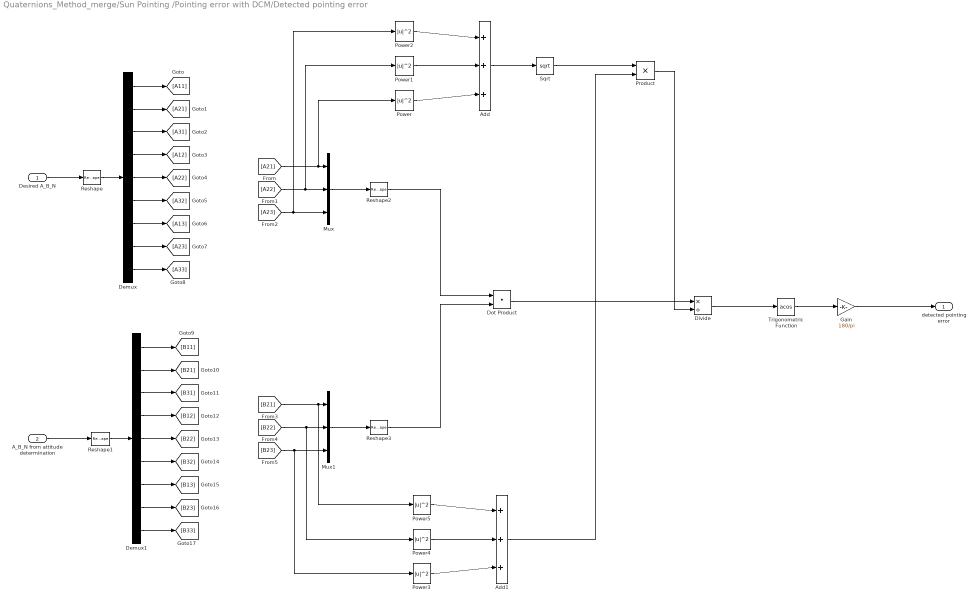
== system Quaternions_Method_merge/Sun Pointing /Pointing error with DCM/Detected pointing error ==
  Desired A_B_N : Inport
  A_B_N from attitude determination : Inport  Port=2
  Add : Sum  Inputs=+|+|+
  Add1 : Sum  Inputs=+|+|+
  Demux : Demux  Outputs=9
  Demux1 : Demux  Outputs=9
  Divide : Product  Inputs=*/
  Dot Product : DotProduct  InputSameDT=on  OutDataTypeStr=Inherit: Inherit via internal rule
  Gain : Gain  Gain=180/pi
  Mux : Mux  Inputs=3
  Mux1 : Mux  Inputs=3
  Power{,1..5} (6 alike) : Math  Operator=magnitude^2  SaturateOnIntegerOverflow=on
  Product : Product
  Reshape{,1..3} (4 alike) : Reshape  OutputDimensionality=Column vector (2-D)
  Sqrt : Sqrt  SaturateOnIntegerOverflow=on
  Trigonometric Function : Trigonometry  Operator=acos
  detected pointing error : Outport
  wires:
  Desired A_B_N/1 -> Reshape/1
  Reshape/1 -> Demux/1
  Demux/1 -> [A11]
  Demux/2 -> [A21]
  Demux/3 -> [A31]
  Demux/4 -> [A12]
  Demux/5 -> [A22]
  Demux/6 -> [A32]
  Demux/7 -> [A13]
  Demux/8 -> [A23]
  Demux/9 -> [A33]
  Demux1/7 -> [B13]
  Demux1/6 -> [B32]
  Demux1/5 -> [B22]
  Demux1/3 -> [B31]
  Demux1/1 -> [B11]
  Demux1/8 -> [B23]
  Demux1/4 -> [B12]
  Reshape1/1 -> Demux1/1
  Demux1/2 -> [B21]
  Demux1/9 -> [B33]
  A_B_N from attitude determination/1 -> Reshape1/1
  [A21] -> Power/1, Mux/1
  [A22] -> Mux/2, Power1/1
  [A23] -> Mux/3, Power2/1
  Mux/1 -> Reshape2/1
  Mux1/1 -> Reshape3/1
  [B22] -> Mux1/2, Power4/1
  [B21] -> Power5/1, Mux1/1
  [B23] -> Mux1/3, Power3/1
  Reshape2/1 -> Dot Product/1
  Reshape3/1 -> Dot Product/2
  Dot Product/1 -> Divide/1
  Power1/1 -> Add/2
  Power2/1 -> Add/1
  Power/1 -> Add/3
  Add/1 -> Sqrt/1
  Sqrt/1 -> Product/1
  Power4/1 -> Add1/2
  Power5/1 -> Add1/1
  Power3/1 -> Add1/3
  Add1/1 -> Product/2
  Product/1 -> Divide/2
  Divide/1 -> Trigonometric Function/1
  Trigonometric Function/1 -> Gain/1
  Gain/1 -> detected pointing error/1

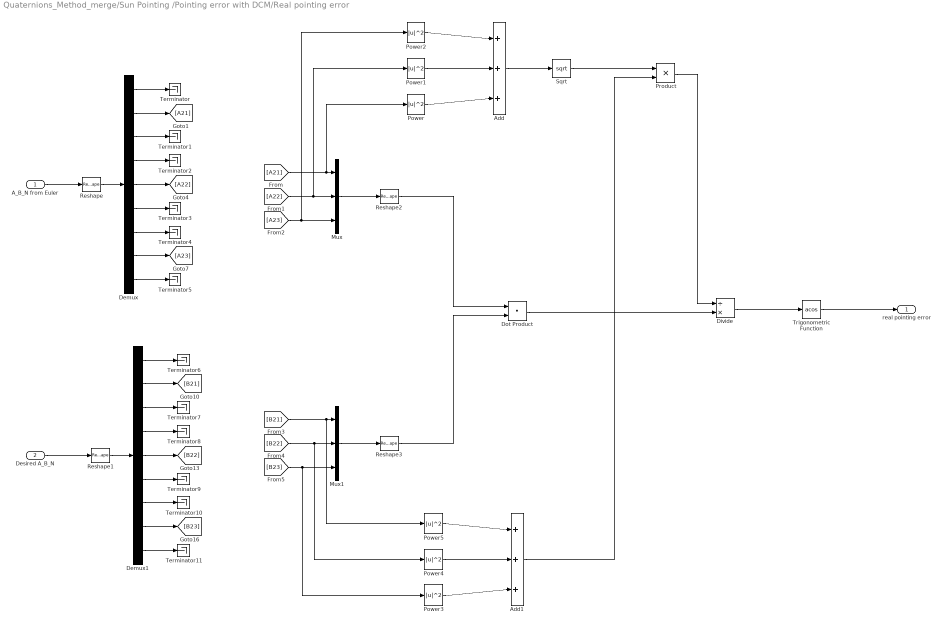
== system Quaternions_Method_merge/Sun Pointing /Pointing error with DCM/Real pointing error ==
  " A_B_N from Euler" : Inport
  Desired A_B_N : Inport  Port=2
  Add : Sum  Inputs=+|+|+
  Add1 : Sum  Inputs=+|+|+
  Demux : Demux  Outputs=9
  Demux1 : Demux  Outputs=9
  Divide : Product  Inputs=/*
  Dot Product : DotProduct  InputSameDT=on  OutDataTypeStr=Inherit: Inherit via internal rule
  Mux : Mux  Inputs=3
  Mux1 : Mux  Inputs=3
  Power{,1..5} (6 alike) : Math  Operator=magnitude^2  SaturateOnIntegerOverflow=on
  Product : Product
  Reshape{,1..3} (4 alike) : Reshape  OutputDimensionality=Column vector (2-D)
  Sqrt : Sqrt  SaturateOnIntegerOverflow=on
  Terminator{,1..11} (12 alike) : Terminator
  Trigonometric Function : Trigonometry  Operator=acos
  real pointing error : Outport
  wires:
  Divide/1 -> Trigonometric Function/1
  Product/1 -> Divide/1
  Add1/1 -> Product/2
  Power3/1 -> Add1/3
  Power5/1 -> Add1/1
  Power4/1 -> Add1/2
  Sqrt/1 -> Product/1
  Add/1 -> Sqrt/1
  Power/1 -> Add/3
  Power2/1 -> Add/1
  Power1/1 -> Add/2
  Dot Product/1 -> Divide/2
  Reshape3/1 -> Dot Product/2
  Reshape2/1 -> Dot Product/1
  [B23] -> Power3/1, Mux1/3
  [B21] -> Mux1/1, Power5/1
  [B22] -> Power4/1, Mux1/2
  Mux1/1 -> Reshape3/1
  Mux/1 -> Reshape2/1
  [A23] -> Power2/1, Mux/3
  [A22] -> Power1/1, Mux/2
  [A21] -> Mux/1, Power/1
  Desired A_B_N/1 -> Reshape1/1
  Demux1/9 -> Terminator11/1
  Demux1/2 -> [B21]
  Reshape1/1 -> Demux1/1
  Demux1/4 -> Terminator8/1
  Demux1/8 -> [B23]
  Demux1/1 -> Terminator6/1
  Demux1/3 -> Terminator7/1
  Demux1/5 -> [B22]
  Demux1/6 -> Terminator9/1
  Demux1/7 -> Terminator10/1
  Demux/9 -> Terminator5/1
  Demux/8 -> [A23]
  Demux/7 -> Terminator4/1
  Demux/6 -> Terminator3/1
  Demux/5 -> [A22]
  Demux/4 -> Terminator2/1
  Demux/3 -> Terminator1/1
  Demux/2 -> [A21]
  Demux/1 -> Terminator/1
  Reshape/1 -> Demux/1
  " A_B_N from Euler"/1 -> Reshape/1
  Trigonometric Function/1 -> real pointing error/1

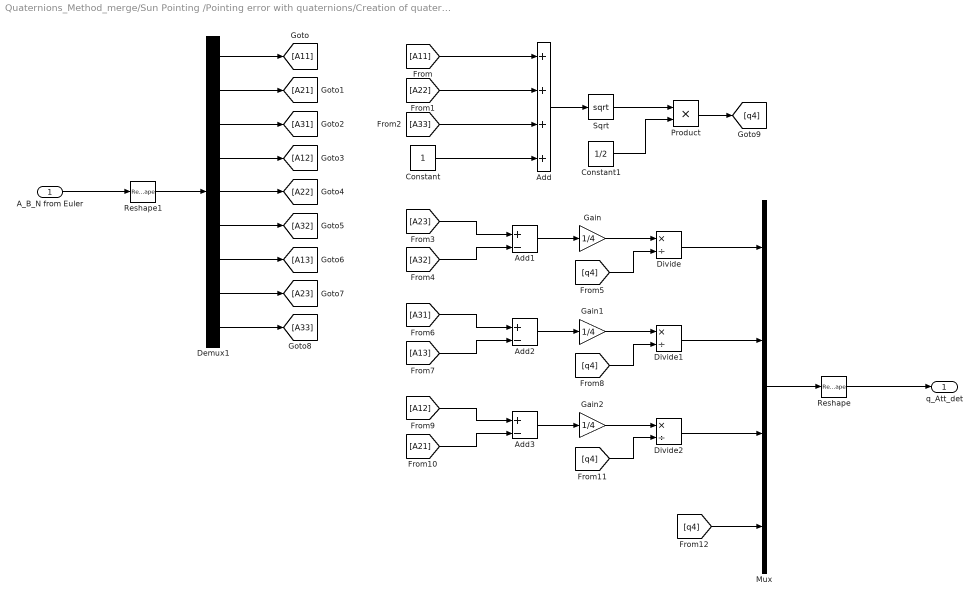
== system Quaternions_Method_merge/Sun Pointing /Pointing error with quaternions/Creation of quaternion ==
  A_B_N from Euler : Inport
  Add : Sum  Inputs=+|+|+|+
  Add1 : Sum  Inputs=+|-
  Add2 : Sum  Inputs=+|-
  Add3 : Sum  Inputs=+|-
  Constant : Constant
  Constant1 : Constant  Value=1/2
  Demux1 : Demux  Outputs=9
  Divide : Product  Inputs=*/
  Divide1 : Product  Inputs=*/
  Divide2 : Product  Inputs=*/
  Gain : Gain  Gain=1/4
  Gain1 : Gain  Gain=1/4
  Gain2 : Gain  Gain=1/4
  Mux : Mux
  Product : Product
  Reshape : Reshape  OutputDimensionality=Column vector (2-D)
  Reshape1 : Reshape  OutputDimensionality=Column vector (2-D)
  Sqrt : Sqrt  SaturateOnIntegerOverflow=on
  q_Att_det : Outport
  wires:
  [q4] -> Mux/4
  [q4] -> Divide/2
  [A12] -> Add3/1
  Gain2/1 -> Divide2/1
  [A21] -> Add3/2
  Add3/1 -> Gain2/1
  Product/1 -> [q4]
  Sqrt/1 -> Product/1
  [q4] -> Divide2/2
  [A11] -> Add/1
  [A31] -> Add2/1
  [A13] -> Add2/2
  Gain1/1 -> Divide1/1
  Add2/1 -> Gain1/1
  [q4] -> Divide1/2
  Add1/1 -> Gain/1
  Add/1 -> Sqrt/1
  Constant1/1 -> Product/2
  [A23] -> Add1/1
  Divide2/1 -> Mux/3
  [A22] -> Add/2
  Constant/1 -> Add/4
  Demux1/4 -> [A12]
  Demux1/2 -> [A21]
  Demux1/3 -> [A31]
  [A32] -> Add1/2
  Demux1/5 -> [A22]
  Demux1/7 -> [A13]
  Demux1/1 -> [A11]
  Gain/1 -> Divide/1
  Divide1/1 -> Mux/2
  Divide/1 -> Mux/1
  Reshape/1 -> q_Att_det/1
  Demux1/9 -> [A33]
  Mux/1 -> Reshape/1
  Demux1/8 -> [A23]
  [A33] -> Add/3
  Demux1/6 -> [A32]
  A_B_N from Euler/1 -> Reshape1/1
  Reshape1/1 -> Demux1/1

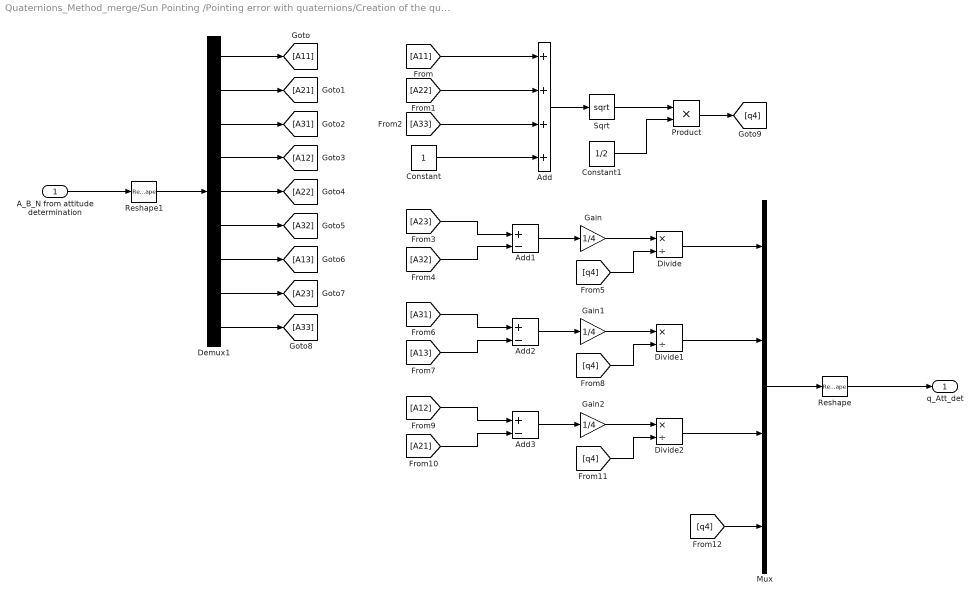
== system Quaternions_Method_merge/Sun Pointing /Pointing error with quaternions/Creation of the quaternion ==
  A_B_N from attitude determination : Inport
  Add : Sum  Inputs=+|+|+|+
  Add1 : Sum  Inputs=+|-
  Add2 : Sum  Inputs=+|-
  Add3 : Sum  Inputs=+|-
  Constant : Constant
  Constant1 : Constant  Value=1/2
  Demux1 : Demux  Outputs=9
  Divide : Product  Inputs=*/
  Divide1 : Product  Inputs=*/
  Divide2 : Product  Inputs=*/
  Gain : Gain  Gain=1/4
  Gain1 : Gain  Gain=1/4
  Gain2 : Gain  Gain=1/4
  Mux : Mux
  Product : Product
  Reshape : Reshape  OutputDimensionality=Column vector (2-D)
  Reshape1 : Reshape  OutputDimensionality=Column vector (2-D)
  Sqrt : Sqrt  SaturateOnIntegerOverflow=on
  q_Att_det : Outport
  wires:
  A_B_N from attitude determination/1 -> Reshape1/1
  Reshape1/1 -> Demux1/1
  Demux1/7 -> [A13]
  Demux1/5 -> [A22]
  Demux1/3 -> [A31]
  Demux1/2 -> [A21]
  Demux1/4 -> [A12]
  Demux1/9 -> [A33]
  Demux1/6 -> [A32]
  Demux1/1 -> [A11]
  Demux1/8 -> [A23]
  [A33] -> Add/3
  [A22] -> Add/2
  [A11] -> Add/1
  Constant/1 -> Add/4
  Add/1 -> Sqrt/1
  Sqrt/1 -> Product/1
  Constant1/1 -> Product/2
  Product/1 -> [q4]
  [A23] -> Add1/1
  [A32] -> Add1/2
  Add1/1 -> Gain/1
  Gain/1 -> Divide/1
  [q4] -> Divide/2
  [q4] -> Divide1/2
  Add2/1 -> Gain1/1
  [A13] -> Add2/2
  Gain1/1 -> Divide1/1
  [A31] -> Add2/1
  [q4] -> Divide2/2
  Add3/1 -> Gain2/1
  [A21] -> Add3/2
  Gain2/1 -> Divide2/1
  [A12] -> Add3/1
  Divide1/1 -> Mux/2
  Divide/1 -> Mux/1
  Divide2/1 -> Mux/3
  [q4] -> Mux/4
  Mux/1 -> Reshape/1
  Reshape/1 -> q_Att_det/1

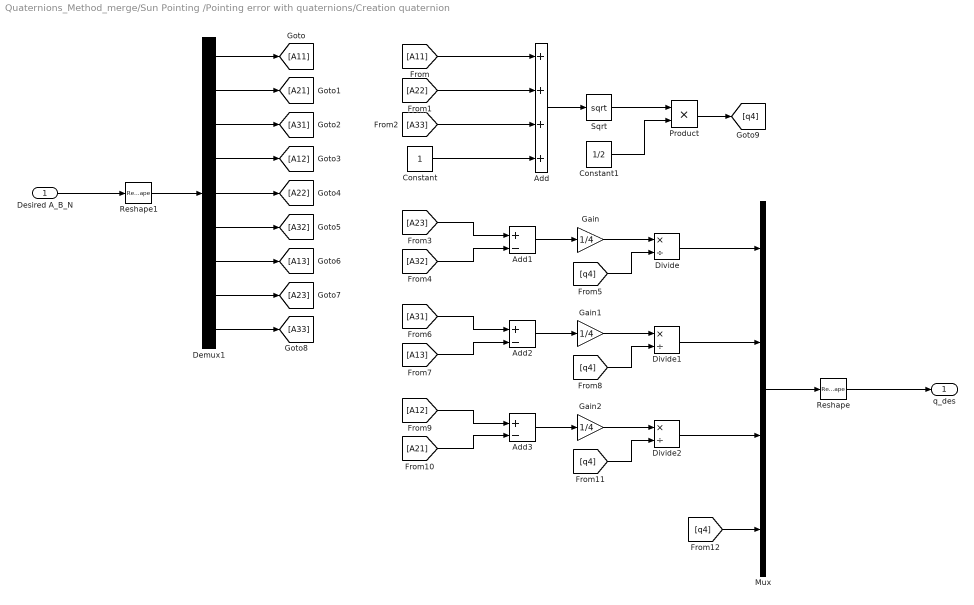
== system Quaternions_Method_merge/Sun Pointing /Pointing error with quaternions/Creation quaternion ==
  Desired A_B_N : Inport
  Add : Sum  Inputs=+|+|+|+
  Add1 : Sum  Inputs=+|-
  Add2 : Sum  Inputs=+|-
  Add3 : Sum  Inputs=+|-
  Constant : Constant
  Constant1 : Constant  Value=1/2
  Demux1 : Demux  Outputs=9
  Divide : Product  Inputs=*/
  Divide1 : Product  Inputs=*/
  Divide2 : Product  Inputs=*/
  Gain : Gain  Gain=1/4
  Gain1 : Gain  Gain=1/4
  Gain2 : Gain  Gain=1/4
  Mux : Mux
  Product : Product
  Reshape : Reshape  OutputDimensionality=Column vector (2-D)
  Reshape1 : Reshape  OutputDimensionality=Column vector (2-D)
  Sqrt : Sqrt  SaturateOnIntegerOverflow=on
  q_des : Outport
  wires:
  [q4] -> Mux/4
  [q4] -> Divide/2
  [A12] -> Add3/1
  Gain2/1 -> Divide2/1
  [A21] -> Add3/2
  Add3/1 -> Gain2/1
  Product/1 -> [q4]
  Sqrt/1 -> Product/1
  [q4] -> Divide2/2
  [A11] -> Add/1
  [A31] -> Add2/1
  [A13] -> Add2/2
  Gain1/1 -> Divide1/1
  Add2/1 -> Gain1/1
  [q4] -> Divide1/2
  Add1/1 -> Gain/1
  Add/1 -> Sqrt/1
  Constant1/1 -> Product/2
  [A23] -> Add1/1
  Divide2/1 -> Mux/3
  [A22] -> Add/2
  Constant/1 -> Add/4
  Demux1/4 -> [A12]
  Demux1/2 -> [A21]
  Demux1/3 -> [A31]
  [A32] -> Add1/2
  Demux1/5 -> [A22]
  Demux1/7 -> [A13]
  Demux1/1 -> [A11]
  Gain/1 -> Divide/1
  Divide1/1 -> Mux/2
  Divide/1 -> Mux/1
  Reshape/1 -> q_des/1
  Demux1/9 -> [A33]
  Mux/1 -> Reshape/1
  Demux1/8 -> [A23]
  [A33] -> Add/3
  Demux1/6 -> [A32]
  Desired A_B_N/1 -> Reshape1/1
  Reshape1/1 -> Demux1/1

== system Quaternions_Method_merge/Sun Pointing /Pointing error with quaternions/Desired attitude ==
  S_N : Inport
  Constant : Constant  Value=0
  Constant1 : Constant  Value=0
  Constant2 : Constant
  Cross Product : matrix_library/Cross Product
      settings: SourceProductBaseCode=SL
  Mux : Mux  Inputs=3
  Reshape : Reshape  OutputDimensionality=Column vector (2-D)
  Reshape1 : Reshape  OutputDimensionality=Customize  OutputDimensions=[3,3]
  Transpose : Math  Operator=transpose  SaturateOnIntegerOverflow=on
  Vector Concatenate : Concatenate  NumInputs=3
  Desired A_B_N : Outport
  wires:
  Constant/1 -> Mux/1
  Constant1/1 -> Mux/2
  Constant2/1 -> Mux/3
  Mux/1 -> Reshape/1
  Reshape/1 -> Cross Product/2, Vector Concatenate/3
  S_N/1 -> Vector Concatenate/2, Cross Product/1
  Cross Product/1 -> Vector Concatenate/1
  Vector Concatenate/1 -> Reshape1/1
  Reshape1/1 -> Transpose/1
  Transpose/1 -> Desired A_B_N/1

== system Quaternions_Method_merge/Enviroment/Magnetic torque /Magnetic torque in body frame/Direction of M field ==
  Clock : Clock
  Constant : Constant  Value=eps
  Constant1 : Constant  Value=w_E
  Mux : Mux  Inputs=3
  Product : Product
  Product1 : Product
  Product2 : Product
  Reshape : Reshape  OutputDimensionality=Column vector (2-D)
  Trigonometric Function : Trigonometry
  Trigonometric Function1 : Trigonometry  Operator=cos
  Trigonometric Function2 : Trigonometry  Operator=cos
  Trigonometric Function3 : Trigonometry
  m_vect : Outport
  wires:
  Constant1/1 -> Product/1
  Clock/1 -> Product/2
  Constant/1 -> Trigonometric Function2/1, Trigonometric Function/1
  Product/1 -> Trigonometric Function3/1, Trigonometric Function1/1
  Trigonometric Function/1 -> Product2/1, Product1/1
  Trigonometric Function1/1 -> Product1/2
  Trigonometric Function3/1 -> Product2/2
  Product1/1 -> Mux/1
  Product2/1 -> Mux/2
  Trigonometric Function2/1 -> Mux/3
  Mux/1 -> Reshape/1
  Reshape/1 -> m_vect/1

== system Quaternions_Method_merge/Enviroment/Solar Radiation Perturbation/Force/creation of the areas of the S//C ==
  note: creation of areas of MB:
      | a=lato corto su asse x del BF; b=lato lungo lungo asse y del BF; h = spessore lungo asse z del BF
  MB : Inport
  Demux : Demux
  Product1 : Product
  Product2 : Product
  Product4 : Product
  Terminator : Terminator
  a*b_1 : Outport
  a*b_2 : Outport  Port=2
  a*h_1 : Outport  Port=3
  a*h_2 : Outport  Port=4
  b*h_1 : Outport  Port=5
  b*h_2 : Outport  Port=6
  wires:
  Demux/4 -> Product4/1, Product2/2
  Demux/3 -> Product1/2, Product4/2
  Demux/2 -> Product1/1, Product2/1
  Product1/1 -> a*b_2/1, a*b_1/1  "a*b"
  Product2/1 -> a*h_1/1, a*h_2/1  "a*h"
  Product4/1 -> b*h_2/1, b*h_1/1  "b*h"
  MB/1 -> Demux/1
  Demux/1 -> Terminator/1
